simulink model "Mdl_DLR"  (R2021b)
settings: Solver=FixedStepAuto  StartTime=0.0  StopTime=10.0  FixedStep=DT_s  RelTol=1e-3
values from neighbouring files (symbols this model uses):
  BEMTPitchMax_deg = -30.0    [DD_Mdl.sldd]    (also in initRotorsimulationNREL5MW.m = -30)
  BladeLength_m = 61.5    [DD_Mdl.sldd]    (also in initRotorsimulationNREL5MW.m)
  BladeMass_kg = 17740.0    [DD_Mdl.sldd]    (also in initRotorsimulationNREL5MW.m = 17740)
  BladePitchMax_deg = 0.0    [DD_Mdl.sldd]    (also in initRotorsimulationNREL5MW.m = 0)
  BladePitchrateNorm_degpers = 3.0    [DD_Mdl.sldd]    (also in initRotorsimulationNREL5MW.m = 3)
  BladePitchrateStop_degpers = 9.0    [DD_Mdl.sldd]    (also in initRotorsimulationNREL5MW.m = 9)
  BladePitchStart_deg = -85.0    [DD_Mdl.sldd]    (also in initRotorsimulationNREL5MW.m = -85)
  BladePrecone_deg = 2.5    [DD_Mdl.sldd]    (also in initRotorsimulationNREL5MW.m)
  BladeTwist_deg = 13.308 13.308 13.308 13.308 13.308 13.308 13.308 13.308 13.308 13.308 13.308 13.308 13.181 12.848 12.192 11.561 11.072 10.792 10.232 9.672 9.11 8.534 7.932 7.321 6.711 6.122 5.546 4.971 4.401 3.834 3.332 2.89 2.503 2.116 1.73 1.342 0.954 0.76 0.574 0.404 0.319 0.253 0.216 0.178 0.14 0.101 0.062 0.023 0.0    [DD_Mdl.sldd]    (also in initRotorsimulationNREL5MW.m = [13.308 13.308 13.308 13.308 13.308 13.308 13.308 13.308 13.)
  cperR = 0.054 0.054 0.056 0.058 0.06 0.061 0.063 0.065 0.067 0.069 0.07 0.072 0.073 0.073 0.073 0.074 0.073 0.072 0.071 0.069 0.068 0.066 0.064 0.062 0.06 0.058 0.056 0.054 0.052 0.05 0.049 0.047 0.045 0.043 0.041 0.039 0.037 0.036 0.035 0.033 0.032 0.03 0.028 0.026 0.024 0.022 0.02 0.018 0.017    [DD_Mdl.sldd]    (also in initRotorsimulationNREL5MW.m = [0.054 0.054 0.056 0.058 0.060 0.061 0.063 0.065 0.067 0.069)
  Cut_OffWindSpeed_mpers = 25.0    [DD_Mdl.sldd]    (also in initRotorsimulationNREL5MW.m = 25)
  DownwashCorrection = 0.26    [DD_Mdl.sldd]    (also in initRotorsimulationNREL5MW.m)
  DownwashModelSwitch = 3.0    [DD_Mdl.sldd]    (also in initRotorsimulationNREL5MW.m = 3)
  drperR = 0.024 0.003 0.016 0.016 0.016 0.016 0.016 0.016 0.016 0.016 0.016 0.016 0.016 0.016 0.016 0.016 0.016 0.016 0.032 0.032 0.032 0.032 0.032 0.032 0.032 0.032 0.032 0.032 0.032 0.032 0.032 0.032 0.032 0.032 0.032 0.032 0.032 0.016 0.016 0.016 0.008 0.008 0.008 0.008 0.008 0.008 0.008 0.008 0.005    [DD_Mdl.sldd]    (also in initRotorsimulationNREL5MW.m = [0.024 0.003 0.016 0.016 0.016 0.016 0.016 0.016 0.016 0.016)
  DT = 0.008    [DD_LPV.sldd]    (also in DD_Mdl.sldd)
  DT_s = 0.008    [DD_Mdl.sldd]    (also in initRotorsimulationNREL5MW.m = 0.01)
  g_mpers_2 = 9.81    [DD_Mdl.sldd]    (also in initRotorsimulationNREL5MW.m)
  GeneratorEfficiency = 0.944    [DD_Mdl.sldd]    (also in initRotorsimulationNREL5MW.m)
  GeneratorOptimalModeGain_Nmper_radpers2 = 2128600    [initRotorsimulationNREL5MW.m]
  HubRadius_m = 1.5    [DD_Mdl.sldd]    (also in initRotorsimulationNREL5MW.m)
  Ki = 0.3    [initRotorsimulationNREL5MW.m]
  Kp = 0.1    [initRotorsimulationNREL5MW.m]
  mpermBl = 0.058 0.008 0.044 0.043 0.042 0.034 0.026 0.024 0.023 0.022 0.023 0.024 0.024 0.023 0.022 0.02 0.02 0.02 0.039 0.038 0.037 0.036 0.034 0.033 0.03 0.029 0.028 0.025 0.023 0.021 0.019 0.018 0.016 0.015 0.012 0.011 0.01 0.005 0.004 0.004 0.002 0.002 0.002 0.002 0.001 0.001 0.001 0.0 0.0    [DD_Mdl.sldd]    (also in initRotorsimulationNREL5MW.m = [0.058 0.008 0.044 0.043 0.042 0.034 0.026 0.024 0.023 0.022)
  nBl = 3.0    [DD_Mdl.sldd]    (also in initRotorsimulationNREL5MW.m = 3)
  nR = 49.0    [DD_Mdl.sldd]    (also in initRotorsimulationNREL5MW.m = length(drperR))
  Overhang_m = 5.0    [DD_Mdl.sldd]    (also in initRotorsimulationNREL5MW.m = 5)
  RatedOmega_RPM = 12.1    [DD_Mdl.sldd]    (also in initRotorsimulationNREL5MW.m)
  RatedWindSpeed_mpers = 11.4    [DD_Mdl.sldd]    (also in initRotorsimulationNREL5MW.m)
  rho_kgperm3 = 1.225    [DD_Mdl.sldd]    (also in initRotorsimulationNREL5MW.m)
  rperR = 0.024 0.027 0.043 0.059 0.075 0.09 0.106 0.122 0.138 0.154 0.17 0.186 0.202 0.217 0.233 0.249 0.265 0.281 0.313 0.344 0.376 0.408 0.44 0.471 0.503 0.535 0.567 0.598 0.63 0.662 0.694 0.725 0.757 0.789 0.821 0.852 0.884 0.9 0.916 0.932 0.94 0.948 0.956 0.963 0.971 0.979 0.987 0.995 1.0    [DD_Mdl.sldd]    (also in initRotorsimulationNREL5MW.m = [0.024 0.027 0.043 0.059 0.075 0.090 0.106 0.122 0.138 0.154)
  Shafttilt_deg = 5.0    [DD_Mdl.sldd]    (also in initRotorsimulationNREL5MW.m = 5)
  TipSpeedLoss = 0.0    [DD_Mdl.sldd]    (also in initRotorsimulationNREL5MW.m = 0)
  TowerDamOnperoff = 0.0    [DD_Mdl.sldd]    (also in initRotorsimulationNREL5MW.m = 0)
  TowerDragCoefficient = 0.35    [DD_Mdl.sldd]    (also in initRotorsimulationNREL5MW.m)
  TowerRadius_m = 1.935    [DD_Mdl.sldd]    (also in initRotorsimulationNREL5MW.m)
  wecs = 3.0    [DD_Mdl.sldd]    (also in DD_Mdl1.sldd = 3.0
libraries: simulink x3
(part 1 of 2)
settings Model: DataDictionary=DD_Mdl.sldd  Creator=ditt_aj  LastModifiedBy=ditt_aj
settings SolverCC: AlgebraicLoopSolver=TrustRegion
settings DebuggingCC: SFMachineParentedDataDiag=warning

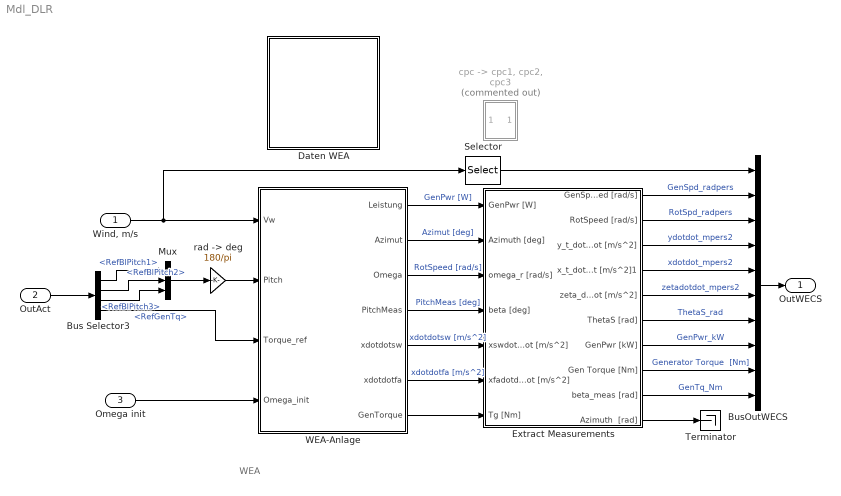
== system Mdl_DLR ==
  note: WEA
  "Wind, m/s" : Inport
  OutAct : Inport  Port=2  OutDataTypeStr=Bus: slBus2
  Omega init : Inport  Port=3
  Bus Selector3 : BusSelector  OutputSignals=RefBlPitch1,RefBlPitch2,RefBlPitch3,RefGenTq
  BusOutWECS : BusCreator  Inputs=10  OutDataTypeStr=Bus: slBus1
  Daten WEA : Subsystem
  Extract Measurements : Subsystem
  Mux : Mux  Inputs=3
  Selector : Selector  InputPortWidth=3  IndexOptions=Index vector (dialog)  Indices=1  OutputSizes=1
  Terminator : Terminator
  WEA-Anlage : Subsystem
  "cpc -> cpc1, cpc2, cpc3" : Subsystem  Commented=on
  "rad -> deg" : Gain  Gain=180/pi
  OutWECS : Outport  OutDataTypeStr=Bus: slBus1
  wires:
  WEA-Anlage/3(Omega) -> Extract Measurements/3("omega_r [rad/s] ")  "RotSpeed [rad/s]"
  WEA-Anlage/2(Azimut) -> Extract Measurements/2(Azimuth [deg])  "Azimut [deg]"
  WEA-Anlage/1(Leistung) -> Extract Measurements/1("GenPwr [W] ")  "GenPwr [W]"
  Omega init/1 -> WEA-Anlage/4(Omega_init)
  WEA-Anlage/4(PitchMeas) -> Extract Measurements/4(beta [deg])  "PitchMeas [deg]"
  WEA-Anlage/5("xdotdotsw ") -> Extract Measurements/5(xswdotdot [m/s^2])  "xdotdotsw [m/s^2]"
  WEA-Anlage/6("xdotdotfa ") -> Extract Measurements/6(xfadotdot [m/s^2])  "xdotdotfa [m/s^2]"
  WEA-Anlage/7(GenTorque) -> Extract Measurements/7(Tg [Nm])
  OutAct/1 -> Bus Selector3/1
  Bus Selector3/4 -> WEA-Anlage/3(Torque_ref)  "<RefGenTq>"
  BusOutWECS/1 -> OutWECS/1
  Extract Measurements/1("GenSpeed [rad/s] ") -> BusOutWECS/2  "GenSpd_radpers"
  Extract Measurements/2(" RotSpeed [rad/s]") -> BusOutWECS/3  "RotSpd_radpers"
  Extract Measurements/3(y_t_dotdot [m/s^2]) -> BusOutWECS/4  "ydotdot_mpers2"
  Extract Measurements/4(x_t_dotdot [m/s^2]1) -> BusOutWECS/5  "xdotdot_mpers2"
  Extract Measurements/5(zeta_dotdot [m/s^2]) -> BusOutWECS/6  "zetadotdot_mpers2"
  Extract Measurements/6(ThetaS [rad]) -> BusOutWECS/7  "ThetaS_rad"
  Extract Measurements/7(GenPwr [kW]) -> BusOutWECS/8  "GenPwr_kW"
  Extract Measurements/8("Gen Torque [Nm]  ") -> BusOutWECS/9  "Generator Torque  [Nm]"
  Extract Measurements/9(beta_meas [rad]) -> BusOutWECS/10  "GenTq_Nm"
  Extract Measurements/10(Azimuth  [rad]) -> Terminator/1
  Mux/1 -> "rad -> deg"/1
  Bus Selector3/1 -> Mux/1  "<RefBlPitch1>"
  Bus Selector3/2 -> Mux/2  "<RefBlPitch2>"
  Bus Selector3/3 -> Mux/3  "<RefBlPitch3>"
  "Wind, m/s"/1 -> WEA-Anlage/1(Vw), Selector/1
  "rad -> deg"/1 -> WEA-Anlage/2(Pitch)
  Selector/1 -> BusOutWECS/1

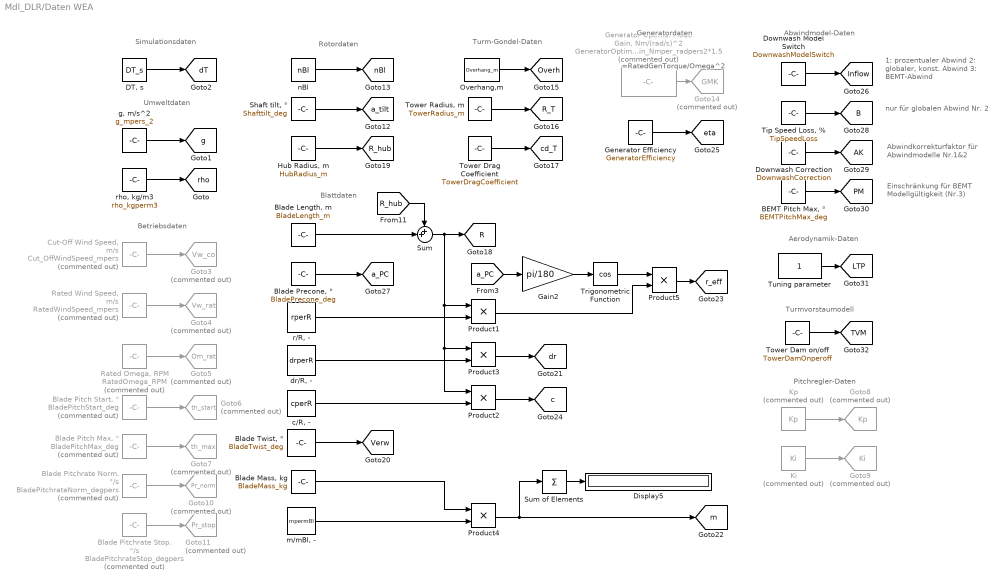
== system Mdl_DLR/Daten WEA ==
  note: Aerodynamik-Daten
  note: Simulationsdaten
  note: Abwindkorrekturfaktor für
      | Abwindmodelle Nr.1&2
  note: Umweltdaten
  note: =RatedGenTorque/Omega^2
  note: Generatordaten
  note: Pitchregler-Daten
  note: Rotordaten
  note: Einschränkung für BEMT
      | Modellgültigkeit (Nr.3)
  note: Betriebsdaten
  note: Abwindmodel-Daten
  note: Turm-Gondel-Daten
  note: nur für globalen Abwind Nr. 2
  note: 1: prozentualer Abwind
      | 2: globaler, konst. Abwind
      | 3: BEMT-Abwind
  note: Turmvorstaumodell
  note: Blattdaten
  "BEMT Pitch Max, °" : Constant  Value=BEMTPitchMax_deg
  "Blade Length, m" : Constant  Value=BladeLength_m
  "Blade Mass, kg" : Constant  Value=BladeMass_kg
  "Blade Pitch Max, °" : Constant  Commented=on  Value=BladePitchMax_deg
  "Blade Pitch Start, °" : Constant  Commented=on  Value=BladePitchStart_deg
  Blade Pitchrate Norm. °/s : Constant  Commented=on  Value=BladePitchrateNorm_degpers
  Blade Pitchrate Stop. °/s : Constant  Commented=on  Value=BladePitchrateStop_degpers
  "Blade Precone, °" : Constant  Value=BladePrecone_deg
  "Blade Twist, °" : Constant  Value=BladeTwist_deg
  "Cut-Off Wind Speed, m/s" : Constant  Commented=on  Value=Cut_OffWindSpeed_mpers
  "DT, s" : Constant  Value=DT_s
  Display5 : Display
  Downwash Correction : Constant  Value=DownwashCorrection
  Downwash Model Switch : Constant  Value=DownwashModelSwitch
  Gain2 : Gain  Gain=pi/180
  Generator Efficiency : Constant  Value=GeneratorEfficiency
  "Generator Optimal Mode Gain, Nm/(rad/s)^2" : Constant  Commented=on  Value=GeneratorOptimalModeGain_Nmper_radpers2*1.5
  Goto10 : Goto  Commented=on  GotoTag=Pr_norm  TagVisibility=global
  Goto11 : Goto  Commented=on  GotoTag=Pr_stop  TagVisibility=global
  Goto14 : Goto  Commented=on  GotoTag=GMK  TagVisibility=global
  Goto3 : Goto  Commented=on  GotoTag=Vw_co  TagVisibility=global
  Goto4 : Goto  Commented=on  GotoTag=Vw_rat  TagVisibility=global
  Goto5 : Goto  Commented=on  GotoTag=Om_rat  TagVisibility=global
  Goto6 : Goto  Commented=on  GotoTag=th_start  TagVisibility=global
  Goto7 : Goto  Commented=on  GotoTag=th_max  TagVisibility=global
  Goto8 : Goto  Commented=on  GotoTag=Kp  TagVisibility=global
  Goto9 : Goto  Commented=on  GotoTag=Ki  TagVisibility=global
  "Hub Radius, m" : Constant  Value=HubRadius_m
  Ki : Constant  Commented=on  Value=Ki
  Kp : Constant  Commented=on  Value=Kp
  Overhang,m : Constant  Value=Overhang_m
  Product{1..5} (5 alike) : Product  RndMeth=Zero
  "Rated Omega, RPM" : Constant  Commented=on  Value=RatedOmega_RPM
  "Rated Wind Speed, m/s" : Constant  Commented=on  Value=RatedWindSpeed_mpers
  "Shaft tilt, °" : Constant  Value=Shafttilt_deg
  Sum : Sum  Inputs=++|
  Sum of Elements : Sum  Inputs=+
  "Tip Speed Loss, %" : Constant  Value=TipSpeedLoss
  Tower Dam on/off : Constant  Value=TowerDamOnperoff
  Tower Drag Coefficient : Constant  Value=TowerDragCoefficient
  "Tower Radius, m" : Constant  Value=TowerRadius_m
  Trigonometric Function : Trigonometry  Operator=cos
  Tuning parameter : Constant
  "c/R, -" : Constant  Value=cperR
  "dr/R, -" : Constant  Value=drperR
  "g, m/s^2" : Constant  Value=g_mpers_2
  "m/mBl, - " : Constant  Value=mpermBl
  nBl : Constant  Value=nBl
  "r/R, -" : Constant  Value=rperR
  "rho, kg/m3" : Constant  Value=rho_kgperm3
  tag scope: AK=global, B=global, Inflow=global, LTP=global, Overh=global, PM=global, R=global, R_T=global, R_hub=global, TVM=global, Verw=global, a_PC=global, a_tilt=global, c=global, cd_T=global, dT=global, dr=global, eta=global, g=global, m=global, nBl=global, r_eff=global, rho=global
  wires:
  Tower Dam on/off/1 -> [TVM]
  Generator Efficiency/1 -> [eta]
  "Blade Precone, °"/1 -> [a_PC]
  "Tower Radius, m"/1 -> [R_T]
  "r/R, -"/1 -> Product1/2
  Downwash Correction/1 -> [AK]
  "DT, s"/1 -> [dT]
  "Blade Pitch Max, °"/1 -> Goto7/1
  [R_hub] -> Sum/1
  "BEMT Pitch Max, °"/1 -> [PM]
  [a_PC] -> Gain2/1
  "Tip Speed Loss, %"/1 -> [B]
  Tuning parameter/1 -> [LTP]
  "g, m/s^2"/1 -> [g]
  "Blade Mass, kg"/1 -> Product4/1
  "Rated Wind Speed, m/s"/1 -> Goto4/1
  Blade Pitchrate Stop. °/s/1 -> Goto11/1
  Sum/1 -> [R], Product1/1, Product3/1, Product2/1
  Downwash Model Switch/1 -> [Inflow]
  Product1/1 -> Product5/2
  Sum of Elements/1 -> Display5/1
  "c/R, -"/1 -> Product2/2
  "Blade Length, m"/1 -> Sum/2
  "Hub Radius, m"/1 -> [R_hub]
  "m/mBl, - "/1 -> Product4/2
  "Shaft tilt, °"/1 -> [a_tilt]
  Product4/1 -> [m], Sum of Elements/1
  Product2/1 -> [c]
  "Blade Twist, °"/1 -> [Verw]
  Tower Drag Coefficient/1 -> [cd_T]
  "dr/R, -"/1 -> Product3/2
  Product3/1 -> [dr]
  Product5/1 -> [r_eff]
  "Blade Pitch Start, °"/1 -> Goto6/1
  Gain2/1 -> Trigonometric Function/1
  "Rated Omega, RPM"/1 -> Goto5/1
  Kp/1 -> Goto8/1
  nBl/1 -> [nBl]
  "Cut-Off Wind Speed, m/s"/1 -> Goto3/1
  Ki/1 -> Goto9/1
  Blade Pitchrate Norm. °/s/1 -> Goto10/1
  "Generator Optimal Mode Gain, Nm/(rad/s)^2"/1 -> Goto14/1
  Trigonometric Function/1 -> Product5/1
  Overhang,m/1 -> [Overh]
  "rho, kg/m3"/1 -> [rho]

== system Mdl_DLR/Extract Measurements ==
  "GenPwr [W] " : Inport
  Azimuth [deg] : Inport  Port=2
  "omega_r [rad/s] " : Inport  Port=3
  beta [deg] : Inport  Port=4
  xswdotdot [m/s^2] : Inport  Port=5
  xfadotdot [m/s^2] : Inport  Port=6
  Tg [Nm] : Inport  Port=7
  "Azimuth: deg -> rad" : Gain  Gain=pi/180
  Demux : Demux  Outputs=3
  Gain6 : Gain  Gain=wecs.Ng
  "GenPwr: W -> kW1" : Gain  Gain=1/1000
  Ground1 : Ground
  "Pitch: deg -> rad" : Gain  Gain=pi/180
  Sum : Sum  Inputs=+-
  Terminator : Terminator
  Terminator1 : Terminator
  "GenSpeed [rad/s] " : Outport  VectorParamsAs1DForOutWhenUnconnected=off
  " RotSpeed [rad/s]" : Outport  Port=2  VectorParamsAs1DForOutWhenUnconnected=off
  y_t_dotdot [m/s^2] : Outport  Port=3  VectorParamsAs1DForOutWhenUnconnected=off
  x_t_dotdot [m/s^2]1 : Outport  Port=4  VectorParamsAs1DForOutWhenUnconnected=off
  zeta_dotdot [m/s^2] : Outport  Port=5  VectorParamsAs1DForOutWhenUnconnected=off
  ThetaS [rad] : Outport  Port=6  VectorParamsAs1DForOutWhenUnconnected=off
  GenPwr [kW] : Outport  Port=7  VectorParamsAs1DForOutWhenUnconnected=off
  "Gen Torque [Nm]  " : Outport  Port=8  VectorParamsAs1DForOutWhenUnconnected=off
  beta_meas [rad] : Outport  Port=9  VectorParamsAs1DForOutWhenUnconnected=off
  Azimuth  [rad] : Outport  Port=10  VectorParamsAs1DForOutWhenUnconnected=off
  wires:
  xfadotdot [m/s^2]/1 -> y_t_dotdot [m/s^2]/1  "y_t_dotdot"
  Gain6/1 -> "GenSpeed [rad/s] "/1  "omega_g [rad/s]"
  Tg [Nm]/1 -> "Gen Torque [Nm]  "/1
  Sum/1 -> ThetaS [rad]/1  "rad"
  "omega_r [rad/s] "/1 -> " RotSpeed [rad/s]"/1, Sum/2, Sum/1, Gain6/1  "GenSpeed [rad/s] LSS"
  Ground1/1 -> zeta_dotdot [m/s^2]/1  "zeta_dotdot"
  xswdotdot [m/s^2]/1 -> x_t_dotdot [m/s^2]1/1  "y_t_dotdot"
  beta [deg]/1 -> "Pitch: deg -> rad"/1  "Pitch [deg]"
  "GenPwr [W] "/1 -> "GenPwr: W -> kW1"/1  "Gen Pwr [W]"
  "GenPwr: W -> kW1"/1 -> GenPwr [kW]/1  "Generator Power [kW]"
  "Azimuth: deg -> rad"/1 -> Azimuth  [rad]/1  "Azimuth [rad]"
  Azimuth [deg]/1 -> "Azimuth: deg -> rad"/1  "Azimuth [deg]"
  "Pitch: deg -> rad"/1 -> Demux/1  "Pitch [rad]"
  Demux/3 -> Terminator/1
  Demux/2 -> Terminator1/1
  Demux/1 -> beta_meas [rad]/1

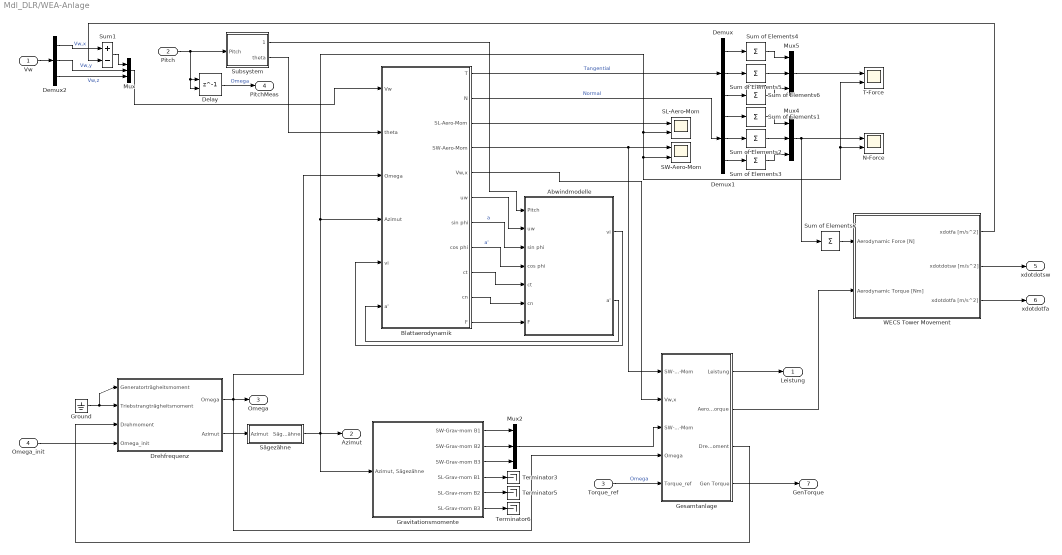
== system Mdl_DLR/WEA-Anlage ==
  Vw : Inport
  Pitch : Inport  Port=2
  Torque_ref : Inport  Port=3
  Omega_init : Inport  Port=4
  Abwindmodelle : Subsystem
  Blattaerodynamik : Subsystem
  Delay : Delay  DelayLength=1  InitialConditionSource=Input port
      settings: InputPortMap=u0,p4
  Demux : Demux  Outputs=3
  Demux1 : Demux  Outputs=3
  Demux2 : Demux  Outputs=3
  Drehfrequenz : Subsystem
  Gesamtanlage : Subsystem
  Gravitationsmomente : Subsystem
  Ground : Ground
  Mux{,2,4..5} (4 alike) : Mux  Inputs=3
  N-Force : Scope  NumInputPorts=2
  SL-Aero-Mom : Scope  NumInputPorts=2
  SW-Aero-Mom : Scope  NumInputPorts=2
  Subsystem : Subsystem
  Sum of Elements{1..7} (7 alike) : Sum  Inputs=+
  Sum1 : Sum  Inputs=+-
  Sägezähne : Subsystem
  T-Force : Scope  NumInputPorts=2
  Terminator3 : Terminator
  Terminator5 : Terminator
  Terminator6 : Terminator
  WECS Tower Movement : Subsystem
  Leistung : Outport  VectorParamsAs1DForOutWhenUnconnected=off
  Azimut : Outport  Port=2  VectorParamsAs1DForOutWhenUnconnected=off
  Omega : Outport  Port=3  VectorParamsAs1DForOutWhenUnconnected=off
  PitchMeas : Outport  Port=4  VectorParamsAs1DForOutWhenUnconnected=off
  "xdotdotsw " : Outport  Port=5  VectorParamsAs1DForOutWhenUnconnected=off
  "xdotdotfa " : Outport  Port=6  VectorParamsAs1DForOutWhenUnconnected=off
  GenTorque : Outport  Port=7  VectorParamsAs1DForOutWhenUnconnected=off
  wires:
  Blattaerodynamik/1(T) -> Demux/1  "Tangential"
  Blattaerodynamik/2(N) -> Demux1/1  "Normal"
  Sägezähne/1(Sägezähne) -> Gravitationsmomente/1("Azimut, Sägezähne"), Blattaerodynamik/4(Azimut), SL-Aero-Mom/2, SW-Aero-Mom/2, N-Force/2, T-Force/2, Azimut/1
  Drehfrequenz/2(Azimut) -> Sägezähne/1(Azimut)
  Blattaerodynamik/4(SW-Aero-Mom) -> Gesamtanlage/1(SW-Aero-Mom), SW-Aero-Mom/1
  Blattaerodynamik/3(SL-Aero-Mom) -> SL-Aero-Mom/1
  Gravitationsmomente/1(SW-Grav-mom B1) -> Mux2/1
  Gravitationsmomente/2(SW-Grav-mom B2) -> Mux2/2
  Gravitationsmomente/3(SW-Grav-mom B3) -> Mux2/3
  Abwindmodelle/1(vi) -> Blattaerodynamik/5(vi)
  Blattaerodynamik/8(cos phi) -> Abwindmodelle/4(cos phi)  "a'"
  Blattaerodynamik/7(sin phi) -> Abwindmodelle/3(sin phi)  "a"
  Blattaerodynamik/10(cn) -> Abwindmodelle/6(cn)
  Blattaerodynamik/9(ct) -> Abwindmodelle/5(ct)
  Abwindmodelle/2(a') -> Blattaerodynamik/6(a')
  Subsystem/2(theta) -> Blattaerodynamik/2(theta)
  Blattaerodynamik/11(F) -> Abwindmodelle/7(F)
  Gravitationsmomente/4(SL-Grav-mom B1) -> Terminator3/1
  Gravitationsmomente/6(SL-Grav-mom B3) -> Terminator6/1
  Gravitationsmomente/5(SL-Grav-mom B2) -> Terminator5/1
  Drehfrequenz/1(Omega) -> Gesamtanlage/4(Omega), Omega/1, Blattaerodynamik/3(Omega)
  Mux2/1 -> Gesamtanlage/3(SW-Grav-Mom)
  Gesamtanlage/1(Leistung) -> Leistung/1
  Gesamtanlage/3(Drehmoment) -> Drehfrequenz/3(Drehmoment)
  Demux1/1 -> Sum of Elements1/1
  Demux1/2 -> Sum of Elements2/1
  Demux1/3 -> Sum of Elements3/1
  Sum of Elements1/1 -> Mux4/1
  Sum of Elements2/1 -> Mux4/2
  Demux/1 -> Sum of Elements4/1
  Demux/2 -> Sum of Elements5/1
  Demux/3 -> Sum of Elements6/1
  Sum of Elements4/1 -> Mux5/1
  Sum of Elements6/1 -> Mux5/3
  Sum of Elements5/1 -> Mux5/2
  Mux5/1 -> T-Force/1
  Blattaerodynamik/5(Vw,x) -> Gesamtanlage/2(Vw,x)
  Blattaerodynamik/6(" uw") -> Abwindmodelle/2(uw)
  Subsystem/1(CPC +IPC) -> Abwindmodelle/1(Pitch)
  Ground/1 -> Drehfrequenz/1(Generatorträgheitsmoment), Drehfrequenz/2(Triebstrangträgheitsmoment)
  Sum of Elements3/1 -> Mux4/3
  Pitch/1 -> Delay/2, Delay/1, Subsystem/1(Pitch)
  Omega_init/1 -> Drehfrequenz/4(Omega_init)
  Delay/1 -> PitchMeas/1  "Omega"
  Mux4/1 -> N-Force/1, Sum of Elements7/1
  Sum of Elements7/1 -> WECS Tower Movement/1(Aerodynamic Force [N])
  Torque_ref/1 -> Gesamtanlage/5(Torque_ref)  "Omega"
  WECS Tower Movement/3(xdotdotfa [m/s^2]) -> "xdotdotfa "/1
  WECS Tower Movement/2(xdotdotsw [m/s^2]) -> "xdotdotsw "/1
  WECS Tower Movement/1(xdotfa [m/s^2]) -> Sum1/2
  Vw/1 -> Demux2/1
  Demux2/1 -> Sum1/1  "Vw,x"
  Sum1/1 -> Mux/1
  Demux2/2 -> Mux/2  "Vw,y"
  Demux2/3 -> Mux/3  "Vw,z"
  Mux/1 -> Blattaerodynamik/1(Vw)
  Gesamtanlage/2(Aero Torque) -> WECS Tower Movement/2(Aerodynamic Torque [Nm])
  Gesamtanlage/4(Gen Torque) -> GenTorque/1

== system Mdl_DLR/cpc -> cpc1, cpc2, cpc3 ==
  beta_ref [rad] : Inport
  Mux : Mux  Inputs=3
  "rad -> deg" : Gain  Gain=180/pi
  "Pitch_ref123 [deg] " : Outport  VectorParamsAs1DForOutWhenUnconnected=off
  wires:
  beta_ref [rad]/1 -> "rad -> deg"/1
  Mux/1 -> "Pitch_ref123 [deg] "/1
  "rad -> deg"/1 -> ?

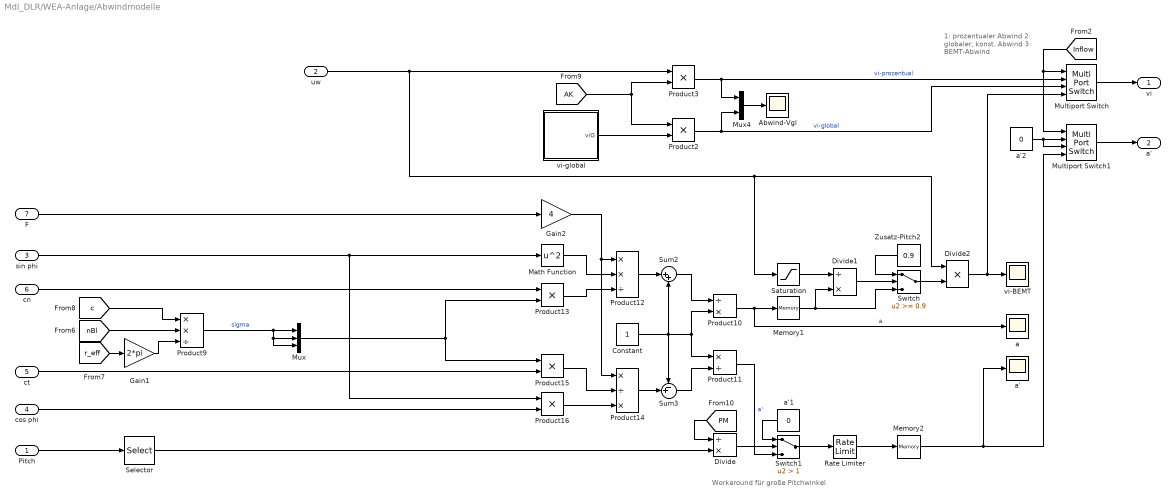
== system Mdl_DLR/WEA-Anlage/Abwindmodelle ==
  note: Workaround für große Pitchwinkel
  note: 1: prozentualer Abwind
      | 2: globaler, konst. Abwind
      | 3: BEMT-Abwind
  Pitch : Inport
  uw : Inport  Port=2
  sin phi : Inport  Port=3
  cos phi : Inport  Port=4
  ct : Inport  Port=5
  cn : Inport  Port=6
  F : Inport  Port=7
  " a " : Scope
  " a' " : Scope
  Abwind-Vgl : Scope
  Constant : Constant
  Divide : Product  Inputs=/*
  Divide1 : Product  Inputs=/*
  Divide2 : Product
  Gain1 : Gain  Gain=2*pi
  Gain2 : Gain  Gain=4
  Math Function : Math  Operator=square  SignedPower=on  SaturateOnIntegerOverflow=on
  Memory1 : Memory
  Memory2 : Memory
  Multiport Switch : MultiPortSwitch  RndMeth=Nearest
  Multiport Switch1 : MultiPortSwitch  RndMeth=Nearest
  Mux : Mux  Inputs=3
  Mux4 : Mux  Inputs=2
  Product10 : Product  Inputs=/*  RndMeth=Zero
  Product11 : Product  Inputs=*/  RndMeth=Zero
  Product12 : Product  Inputs=**/  RndMeth=Zero
  Product{2..3,13,15..16} (5 alike) : Product  RndMeth=Zero
  Product14 : Product  Inputs=*/*  RndMeth=Zero
  Product9 : Product  Inputs=**/  RndMeth=Zero
  Rate Limiter : RateLimiter  SampleTimeMode=inherited
  Saturation : Saturate  UpperLimit=inf  LowerLimit=0.01
  Selector : Selector  InputPortWidth=3  IndexOptions=Index vector (dialog)  Indices=1  OutputSizes=1
  Sum2 : Sum  Inputs=|++
  Sum3 : Sum  Inputs=-+|
  Switch : Switch  Threshold=0.9
  Switch1 : Switch  Criteria=u2 > Threshold  Threshold=1
  Zusatz-Pitch2 : Constant  Value=0.9
  a'1 : Constant  Value=0
  a'2 : Constant  Value=0
  vi-BEMT : Scope
  vi-global : Subsystem
  vi : Outport  VectorParamsAs1DForOutWhenUnconnected=off
  a' : Outport  Port=2  VectorParamsAs1DForOutWhenUnconnected=off
  wires:
  vi-global/1(viG) -> Product2/2
  Product2/1 -> Mux4/2, Multiport Switch/3  "vi-global"
  Saturation/1 -> Divide1/1
  Zusatz-Pitch2/1 -> Switch/1
  Memory1/1 -> Divide1/2, Switch/3
  Switch/1 -> Divide2/2
  Divide1/1 -> Switch/2
  Divide2/1 -> vi-BEMT/1, Multiport Switch/4
  [Inflow] -> Multiport Switch/1, Multiport Switch1/1
  Mux4/1 -> Abwind-Vgl/1
  Product3/1 -> Mux4/1, Multiport Switch/2  "vi-prozentual"
  uw/1 -> Saturation/1, Divide2/1, Product3/1
  Multiport Switch/1 -> vi/1
  cos phi/1 -> Product16/2
  sin phi/1 -> Math Function/1, Product16/1
  Constant/1 -> Sum3/1, Sum2/2, Product11/1, Product10/2
  Math Function/1 -> Product12/2
  Product13/1 -> Product12/3
  cn/1 -> Product13/1
  Product16/1 -> Product14/3
  ct/1 -> Product15/2
  Product12/1 -> Sum2/1
  Product14/1 -> Sum3/2
  Sum2/1 -> Product10/1
  Sum3/1 -> Product11/2
  Product10/1 -> Memory1/1, " a "/1  "a"
  Product11/1 -> Switch1/3  "a'"
  [c] -> Product9/1
  [nBl] -> Product9/2
  [r_eff] -> Gain1/1
  Gain1/1 -> Product9/3
  a'2/1 -> Multiport Switch1/2, Multiport Switch1/3
  Multiport Switch1/1 -> a'/1
  F/1 -> Gain2/1
  Gain2/1 -> Product12/1, Product14/1
  Product15/1 -> Product14/2
  Pitch/1 -> Selector/1
  Divide/1 -> Switch1/2
  a'1/1 -> Switch1/1
  [PM] -> Divide/1
  Switch1/1 -> Rate Limiter/1
  Rate Limiter/1 -> Memory2/1
  Memory2/1 -> " a' "/1, Multiport Switch1/4
  [AK] -> Product3/2, Product2/1
  Selector/1 -> Divide/2
  Product9/1 -> Mux/3, Mux/2, Mux/1  "sigma"
  Mux/1 -> Product15/1, Product13/2

== system Mdl_DLR/WEA-Anlage/Blattaerodynamik ==
  Vw : Inport
  theta : Inport  Port=2
  Omega : Inport  Port=3
  Azimut : Inport  Port=4
  vi : Inport  Port=5
  a' : Inport  Port=6
  Anströmung : Subsystem
  Beiwerte1 : Subsystem
  Beiwerte2 : Subsystem
  Blattbiegemomente : Subsystem
  Gain5 : Gain  Gain=pi/180
  Komponenten für BEMT : Subsystem
  Normal-/Tangentialkraft : Subsystem
  Tip&Hub-Loss-Faktor : Subsystem
  T : Outport  VectorParamsAs1DForOutWhenUnconnected=off
  N : Outport  Port=2  VectorParamsAs1DForOutWhenUnconnected=off
  SL-Aero-Mom : Outport  Port=3  VectorParamsAs1DForOutWhenUnconnected=off
  SW-Aero-Mom : Outport  Port=4  VectorParamsAs1DForOutWhenUnconnected=off
  Vw,x : Outport  Port=5  VectorParamsAs1DForOutWhenUnconnected=off
  " uw" : Outport  Port=6  VectorParamsAs1DForOutWhenUnconnected=off
  sin phi : Outport  Port=7  VectorParamsAs1DForOutWhenUnconnected=off
  cos phi : Outport  Port=8  VectorParamsAs1DForOutWhenUnconnected=off
  ct : Outport  Port=9  VectorParamsAs1DForOutWhenUnconnected=off
  cn : Outport  Port=10  VectorParamsAs1DForOutWhenUnconnected=off
  F : Outport  Port=11  VectorParamsAs1DForOutWhenUnconnected=off
  wires:
  Beiwerte2/1(cl) -> Normal-/Tangentialkraft/1(cl)
  Beiwerte2/2(cd) -> Normal-/Tangentialkraft/2(cd)
  Anströmung/2(phi) -> Normal-/Tangentialkraft/3("phi, rad")
  Anströmung/3(V^2) -> Normal-/Tangentialkraft/4(V^2)
  Vw/1 -> Anströmung/2(Vw)
  Omega/1 -> Anströmung/4(Omega)
  Normal-/Tangentialkraft/1(T) -> T/1, Blattbiegemomente/1(T)
  Normal-/Tangentialkraft/2(N) -> N/1, Blattbiegemomente/2(N)
  Komponenten für BEMT/1(sin phi) -> sin phi/1, Tip&Hub-Loss-Faktor/1(sin phi)
  theta/1 -> Anströmung/1(theta)
  vi/1 -> Anströmung/3(vi)
  Komponenten für BEMT/3(ct) -> ct/1
  Komponenten für BEMT/4(cn) -> cn/1
  a'/1 -> Anströmung/5(a')
  Anströmung/1(alf_eff) -> Beiwerte2/1("alf_eff, rad")
  Tip&Hub-Loss-Faktor/1(F) -> F/1
  Azimut/1 -> Gain5/1
  Gain5/1 -> Anströmung/6(Azimut)
  Anströmung/5(uw) -> " uw"/1
  Anströmung/4(Vw,x) -> Vw,x/1
  Anströmung/6(phi BEMT) -> Komponenten für BEMT/1("phi, BEMT")
  Komponenten für BEMT/2(cos phi) -> cos phi/1
  Anströmung/7(alf_eff_BEMT) -> Beiwerte1/1("alf_eff, rad")
  Beiwerte1/1(cl) -> Komponenten für BEMT/2(cl)
  Beiwerte1/2(cd) -> Komponenten für BEMT/3(cd)
  Blattbiegemomente/1(SW-Aero-Mom) -> SW-Aero-Mom/1
  Blattbiegemomente/2(SL-Aero-Mom) -> SL-Aero-Mom/1

== system Mdl_DLR/WEA-Anlage/Drehfrequenz ==
  note: Omega = Omega0 + dOm/dt*t
  note: Psi = Psi0 + Omega0*t + 1/2*dOm/dt*t^2
  note: Rotorträgheits-
      | moment
  Generatorträgheitsmoment : Inport
  Triebstrangträgheitsmoment : Inport  Port=2
  Drehmoment : Inport  Port=3
  Omega_init : Inport  Port=4
  Azimut1 : Scope
  Delay : Delay  DelayLength=1  InitialConditionSource=Input port
      settings: InputPortMap=u0,p4
  Delay1 : Delay  DelayLength=1  InitialConditionSource=Input port
      settings: InputPortMap=u0,p4
  Divide : Product  Inputs=*/
  Gain : Gain  Gain=1/2
  Gain4 : Gain  Gain=180/pi
  Math Function : Math  Operator=square  SignedPower=on  SaturateOnIntegerOverflow=on
  Math Function5 : Math  Operator=square  SignedPower=on  SaturateOnIntegerOverflow=on
  Memory2 : Memory
  Omega1 : Scope
  Product1 : Product  RndMeth=Zero
  Product2 : Product  RndMeth=Zero
  Product3 : Product  RndMeth=Zero
  Product4 : Product  Inputs=3  RndMeth=Zero
  Sum of Elements : Sum  Inputs=+
  Sum1 : Sum  Inputs=+++
  Sum2 : Sum  Inputs=++|
  Sum6 : Sum  Inputs=++|
  Sum7 : Sum  Inputs=+|+
  Trägheitsmoment : Display
      settings: Decimation=100
  Omega : Outport  VectorParamsAs1DForOutWhenUnconnected=off
  Azimut : Outport  Port=2  VectorParamsAs1DForOutWhenUnconnected=off
  wires:
  Drehmoment/1 -> Divide/1
  [dT] -> Product2/2, Product1/2, Math Function/1
  Divide/1 -> Gain/1, Product2/1  "dOm/dt"
  Sum2/1 -> Delay1/1, Delay/1, Product1/1  "Omega"
  Delay1/1 -> Sum2/1
  Product2/1 -> Sum2/2
  Sum6/1 -> Memory2/1, Azimut/1, Gain4/1  "Azimut"
  Memory2/1 -> Sum6/1
  Gain/1 -> Product3/2
  Math Function/1 -> Product3/1
  Product1/1 -> Sum7/1
  Product3/1 -> Sum7/2
  Sum7/1 -> Sum6/2
  Delay/1 -> Omega/1, Omega1/1  "Omega"
  [m] -> Product4/3
  Math Function5/1 -> Product4/2
  Product4/1 -> Sum of Elements/1
  [nBl] -> Product4/1
  [r_eff] -> Math Function5/1
  Sum of Elements/1 -> Sum1/2
  Generatorträgheitsmoment/1 -> Sum1/1
  Triebstrangträgheitsmoment/1 -> Sum1/3
  Sum1/1 -> Trägheitsmoment/1, Divide/2
  Gain4/1 -> Azimut1/1  "Azimut"
  Omega_init/1 -> Delay1/2, Delay/2

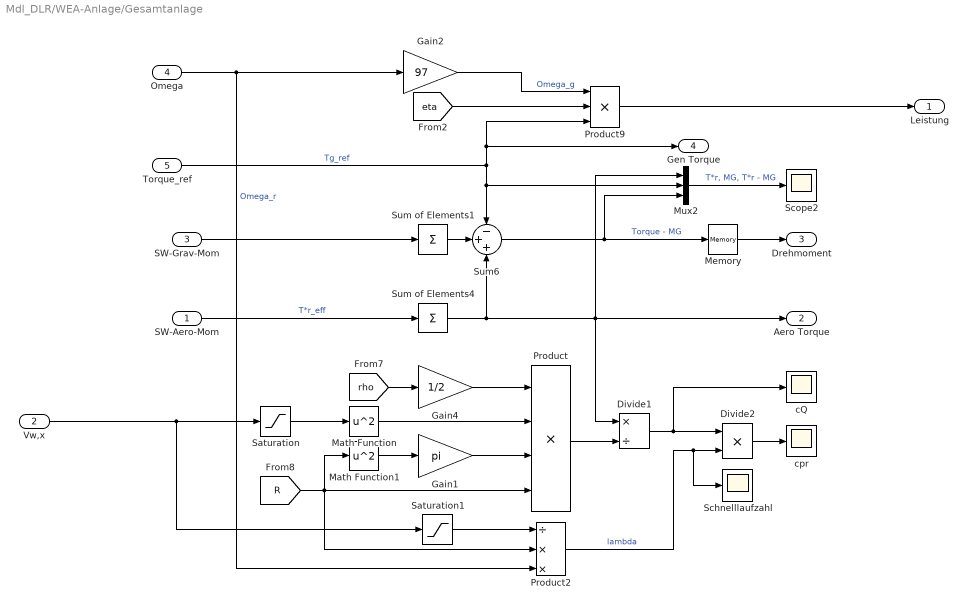
== system Mdl_DLR/WEA-Anlage/Gesamtanlage ==
  SW-Aero-Mom : Inport
  Vw,x : Inport  Port=2
  SW-Grav-Mom : Inport  Port=3
  Omega : Inport  Port=4
  Torque_ref : Inport  Port=5
  Divide1 : Product  Inputs=*/
  Divide2 : Product
  Gain1 : Gain  Gain=pi
  Gain2 : Gain  Gain=97
  Gain4 : Gain  Gain=1/2
  Math Function : Math  Operator=square  SignedPower=on  SaturateOnIntegerOverflow=on
  Math Function1 : Math  Operator=square  SignedPower=on  SaturateOnIntegerOverflow=on
  Memory : Memory
  Mux2 : Mux  Inputs=3
  Product : Product  Inputs=4  RndMeth=Zero
  Product2 : Product  Inputs=/**  RndMeth=Zero
  Product9 : Product  Inputs=3  RndMeth=Zero
  Saturation : Saturate  UpperLimit=inf  LowerLimit=0.1
  Saturation1 : Saturate  UpperLimit=inf  LowerLimit=0.1
  Schnelllaufzahl : Scope
  Scope2 : Scope
  Sum of Elements1 : Sum  Inputs=+
  Sum of Elements4 : Sum  Inputs=+
  Sum6 : Sum  Inputs=-++
  cQ : Scope
  cpr : Scope
  Leistung : Outport  VectorParamsAs1DForOutWhenUnconnected=off
  Aero Torque : Outport  Port=2  VectorParamsAs1DForOutWhenUnconnected=off
  Drehmoment : Outport  Port=3  VectorParamsAs1DForOutWhenUnconnected=off
  Gen Torque : Outport  Port=4  VectorParamsAs1DForOutWhenUnconnected=off
  wires:
  Product2/1 -> Divide2/2, Schnelllaufzahl/1  "lambda"
  Divide2/1 -> cpr/1
  Math Function/1 -> Product/2
  [R] -> Math Function1/1, Product/4, Product2/2
  Math Function1/1 -> Gain1/1
  Gain4/1 -> Product/1
  Gain1/1 -> Product/3
  Product/1 -> Divide1/2
  Divide1/1 -> Divide2/1, cQ/1
  Sum of Elements4/1 -> Sum6/3, Divide1/1, Mux2/1, Aero Torque/1
  [rho] -> Gain4/1
  Saturation/1 -> Math Function/1
  Mux2/1 -> Scope2/1  "T*r, MG, T*r - MG"
  Sum6/1 -> Mux2/3, Memory/1  "Torque - MG"
  SW-Grav-Mom/1 -> Sum of Elements1/1
  [eta] -> Product9/2
  Omega/1 -> Gain2/1, Product2/3  "Omega_r"
  SW-Aero-Mom/1 -> Sum of Elements4/1  "T*r_eff"
  Vw,x/1 -> Saturation1/1, Saturation/1
  Saturation1/1 -> Product2/1
  Sum of Elements1/1 -> Sum6/2
  Memory/1 -> Drehmoment/1
  Torque_ref/1 -> Mux2/2, Sum6/1, Gen Torque/1, Product9/3  "Tg_ref"
  Product9/1 -> Leistung/1
  Gain2/1 -> Product9/1  "Omega_g"

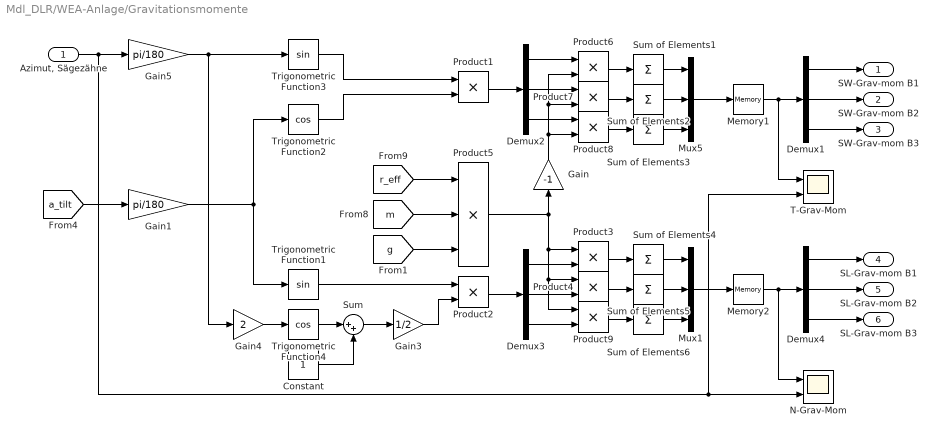
== system Mdl_DLR/WEA-Anlage/Gravitationsmomente ==
  "Azimut, Sägezähne" : Inport
  Constant : Constant
  Demux{1..4} (4 alike) : Demux  Outputs=3
  Gain : Gain  Gain=-1
  Gain1 : Gain  Gain=pi/180
  Gain3 : Gain  Gain=1/2
  Gain4 : Gain  Gain=2
  Gain5 : Gain  Gain=pi/180
  Memory1 : Memory
  Memory2 : Memory
  Mux1 : Mux  Inputs=3
  Mux5 : Mux  Inputs=3
  N-Grav-Mom : Scope  NumInputPorts=2
  Product{1..4,6..9} (8 alike) : Product  RndMeth=Zero
  Product5 : Product  Inputs=3  RndMeth=Zero
  Sum : Sum  Inputs=|++
  Sum of Elements{1..6} (6 alike) : Sum  Inputs=+
  T-Grav-Mom : Scope  NumInputPorts=2
  Trigonometric Function1 : Trigonometry
  Trigonometric Function2 : Trigonometry  Operator=cos
  Trigonometric Function3 : Trigonometry
  Trigonometric Function4 : Trigonometry  Operator=cos
  SW-Grav-mom B1 : Outport  VectorParamsAs1DForOutWhenUnconnected=off
  SW-Grav-mom B2 : Outport  Port=2  VectorParamsAs1DForOutWhenUnconnected=off
  SW-Grav-mom B3 : Outport  Port=3  VectorParamsAs1DForOutWhenUnconnected=off
  SL-Grav-mom B1 : Outport  Port=4  VectorParamsAs1DForOutWhenUnconnected=off
  SL-Grav-mom B2 : Outport  Port=5  VectorParamsAs1DForOutWhenUnconnected=off
  SL-Grav-mom B3 : Outport  Port=6  VectorParamsAs1DForOutWhenUnconnected=off
  wires:
  Gain5/1 -> Trigonometric Function3/1, Gain4/1
  Product5/1 -> Gain/1, Product3/1, Product4/1, Product9/1
  "Azimut, Sägezähne"/1 -> Gain5/1, N-Grav-Mom/2, T-Grav-Mom/2
  Memory1/1 -> Demux1/1, T-Grav-Mom/1
  Product6/1 -> Sum of Elements1/1
  Sum of Elements1/1 -> Mux5/1
  Product7/1 -> Sum of Elements2/1
  Product8/1 -> Sum of Elements3/1
  Sum of Elements2/1 -> Mux5/2
  Sum of Elements3/1 -> Mux5/3
  Demux2/1 -> Product6/1
  Demux2/2 -> Product7/1
  Demux2/3 -> Product8/1
  Mux5/1 -> Memory1/1
  [r_eff] -> Product5/1
  [m] -> Product5/2
  Demux1/1 -> SW-Grav-mom B1/1
  Demux1/2 -> SW-Grav-mom B2/1
  Demux1/3 -> SW-Grav-mom B3/1
  [g] -> Product5/3
  Gain/1 -> Product6/2, Product7/2, Product8/2
  Trigonometric Function4/1 -> Sum/1
  Sum/1 -> Gain3/1
  Constant/1 -> Sum/2
  Gain3/1 -> Product2/2
  [a_tilt] -> Gain1/1
  Gain1/1 -> Trigonometric Function2/1, Trigonometric Function1/1
  Trigonometric Function3/1 -> Product1/1
  Trigonometric Function2/1 -> Product1/2
  Product1/1 -> Demux2/1
  Gain4/1 -> Trigonometric Function4/1
  Trigonometric Function1/1 -> Product2/1
  Product2/1 -> Demux3/1
  Memory2/1 -> Demux4/1, N-Grav-Mom/1
  Product3/1 -> Sum of Elements4/1
  Sum of Elements4/1 -> Mux1/1
  Product4/1 -> Sum of Elements5/1
  Product9/1 -> Sum of Elements6/1
  Sum of Elements5/1 -> Mux1/2
  Sum of Elements6/1 -> Mux1/3
  Mux1/1 -> Memory2/1
  Demux4/1 -> SL-Grav-mom B1/1
  Demux4/2 -> SL-Grav-mom B2/1
  Demux4/3 -> SL-Grav-mom B3/1
  Demux3/3 -> Product9/2
  Demux3/2 -> Product4/2
  Demux3/1 -> Product3/2

== system Mdl_DLR/WEA-Anlage/Subsystem ==
  Pitch : Inport
  Add1 : Sum  Inputs=+-
  Add2 : Sum  Inputs=+-
  Add3 : Sum  Inputs=+-
  Demux : Demux  Outputs=3
  Gain : Gain  Gain=-1
  Gain1 : Gain  Gain=-1
  Mux : Mux  Inputs=3
  CPC +IPC : Outport  VectorParamsAs1DForOutWhenUnconnected=off
  theta : Outport  Port=2  VectorParamsAs1DForOutWhenUnconnected=off
  wires:
  [Verw] -> Gain/1  "Verw."
  Add1/1 -> Mux/1  "radialer Blattsteuerwinkel"
  Pitch/1 -> Gain1/1, Demux/1  "Pitch"
  Demux/1 -> Add1/2
  Demux/2 -> Add2/2
  Demux/3 -> Add3/2
  Add2/1 -> Mux/2  "radialer Blattsteuerwinkel"
  Add3/1 -> Mux/3  "radialer Blattsteuerwinkel"
  Mux/1 -> theta/1
  Gain/1 -> Add1/1, Add3/1, Add2/1
  Gain1/1 -> CPC +IPC/1

== system Mdl_DLR/WEA-Anlage/Sägezähne ==
  Azimut : Inport
  Add4 : Sum
  Add5 : Sum
  Azimute : Scope
  Gain4 : Gain  Gain=180/pi
  Gain6 : Gain  Gain=2
  Generator- moment1 : Constant  Value=-120
  Grad : Constant  Value=0
  Grad1 : Constant  Value=360
  Memory1 : Memory
  Memory2 : Memory
  Memory4 : Memory
  Mux4 : Mux  Inputs=3
  Sum2 : Sum  Inputs=|+-
  Sum3 : Sum  Inputs=|++
  Sum4 : Sum  Inputs=+|+
  Sum5 : Sum  Inputs=|+-
  Switch : Switch  Threshold=360
  Sägezähne : Outport  VectorParamsAs1DForOutWhenUnconnected=off
  wires:
  Grad/1 -> Switch/3
  Grad1/1 -> Switch/1
  Gain4/1 -> Sum2/1, Sum5/1, Memory4/1  "Azimut"
  Switch/1 -> Sum3/1
  Sum2/1 -> Memory1/1, Mux4/1, Add4/1, Add5/1  "Azimut"
  Sum3/1 -> Memory2/1, Sum2/2  "Omega"
  Memory2/1 -> Sum3/2
  Sum4/1 -> Switch/2
  Sum5/1 -> Sum4/2
  Memory4/1 -> Sum5/2
  Azimut/1 -> Gain4/1
  Memory1/1 -> Sum4/1
  Generator- moment1/1 -> Add4/2, Gain6/1
  Add4/1 -> Mux4/2
  Mux4/1 -> Sägezähne/1, Azimute/1  "Azimut"
  Add5/1 -> Mux4/3
  Gain6/1 -> Add5/2

== system Mdl_DLR/WEA-Anlage/WECS Tower Movement ==
  note: Tower Fore-Aft Motion
  note: Tower Side-By-Side Motion
  Aerodynamic Force [N] : Inport
  Aerodynamic Torque [Nm] : Inport  Port=2
  Gain : Gain  Gain=wecs.Btsw/wecs.mt
  Gain1 : Gain  Gain=wecs.Ktsw/wecs.mt
  Gain10 : Gain  Gain=3/(2*wecs.H)
  Gain{4,6,8,14} (4 alike) : Gain  Gain=DT
  Gain2 : Gain  Gain=wecs.Bt/wecs.mt
  Gain3 : Gain  Gain=wecs.Kt/wecs.mt
  Gain5 : Gain  Gain=1/wecs.mt
  Gain7 : Gain  Gain=1/wecs.mt
  Memory{1..4} (4 alike) : Memory
  Sum : Sum  Inputs=+--
  Sum{1,3..5} (4 alike) : Sum
  Sum2 : Sum  Inputs=+--
  xdotfa [m/s^2] : Outport  VectorParamsAs1DForOutWhenUnconnected=off
  xdotdotsw [m/s^2] : Outport  Port=2  VectorParamsAs1DForOutWhenUnconnected=off
  xdotdotfa [m/s^2] : Outport  Port=3  VectorParamsAs1DForOutWhenUnconnected=off
  wires:
  Memory4/1 -> Gain6/1, xdotfa [m/s^2]/1, Sum4/2, Gain2/1  "xdotfa"
  Sum2/1 -> Gain8/1, xdotdotfa [m/s^2]/1  "xdotdotfa"
  Gain5/1 -> Sum2/1
  Gain2/1 -> Sum2/3
  Memory2/1 -> Sum3/2, Gain3/1  "xfa"
  Gain3/1 -> Sum2/2
  Aerodynamic Force [N]/1 -> Gain5/1
  Gain/1 -> Sum/3
  Gain1/1 -> Sum/2
  Gain7/1 -> Sum/1
  Memory1/1 -> Gain/1, Sum1/2, Gain14/1  "xdotss"
  Memory3/1 -> Gain1/1, Sum5/2  "xss"
  Gain10/1 -> Gain7/1  "xdotdotss"
  Aerodynamic Torque [Nm]/1 -> Gain10/1
  Sum5/1 -> Memory3/1  "xdotdotss"
  Gain14/1 -> Sum5/1
  Sum/1 -> xdotdotsw [m/s^2]/1, Gain4/1  "xdotss"
  Sum1/1 -> Memory1/1  "xdotdotss"
  Gain4/1 -> Sum1/1
  Sum3/1 -> Memory2/1  "xdotdotss"
  Gain6/1 -> Sum3/1
  Gain8/1 -> Sum4/1
  Sum4/1 -> Memory4/1  "xdotdotss"

== system Mdl_DLR/WEA-Anlage/Abwindmodelle/vi-global ==
  Abs : Abs
  B1 : Constant  Value=100
  Divide : Product  Inputs=**/
  Divide1 : Product  Inputs=*/
  Divide2 : Product  Inputs=/*
  Divide3 : Product
  Gain : Gain  Gain=2
  Gain1 : Gain  Gain=pi
  Math Function : Math  Operator=square  SignedPower=on  SaturateOnIntegerOverflow=on
  Math Function1 : Math  Operator=sqrt  SignedPower=on  SaturateOnIntegerOverflow=on
  Math Function2 : Math  Operator=square  SignedPower=on  SaturateOnIntegerOverflow=on
  Math Function3 : Math  Operator=square  SignedPower=on  SaturateOnIntegerOverflow=on
  Memory5 : Memory
  Product : Product  Inputs=3  RndMeth=Zero
  Sign : Signum
  Sum : Sum  Inputs=|++
  Sum of Elements : Sum  Inputs=+
  Sum1 : Sum  Inputs=|+-
  Sum2 : Sum  Inputs=|+-
  ra/R : Constant  Value=0.1
  viG : Outport  VectorParamsAs1DForOutWhenUnconnected=off
  wires:
  Gain/1 -> Product/1
  Math Function/1 -> Gain1/1
  Gain1/1 -> Product/2
  Product/1 -> Divide/3
  Divide/1 -> Abs/1, Sign/1
  Sum of Elements/1 -> Divide/1
  [B] -> Sum2/2, Divide1/1
  B1/1 -> Divide1/2, Sum2/1, Divide2/1
  Divide1/1 -> Sum/1
  Sum/1 -> Math Function2/1
  Math Function2/1 -> Sum1/2
  Divide2/1 -> Math Function3/1
  Math Function3/1 -> Sum1/1
  Sum1/1 -> Product/3
  [nBl] -> Divide/2
  [N] -> Sum of Elements/1
  [rho] -> Gain/1
  [R] -> Math Function/1
  ra/R/1 -> Sum/2
  Sum2/1 -> Divide2/2
  Memory5/1 -> viG/1
  Abs/1 -> Math Function1/1
  Math Function1/1 -> Divide3/1
  Sign/1 -> Divide3/2
  Divide3/1 -> Memory5/1

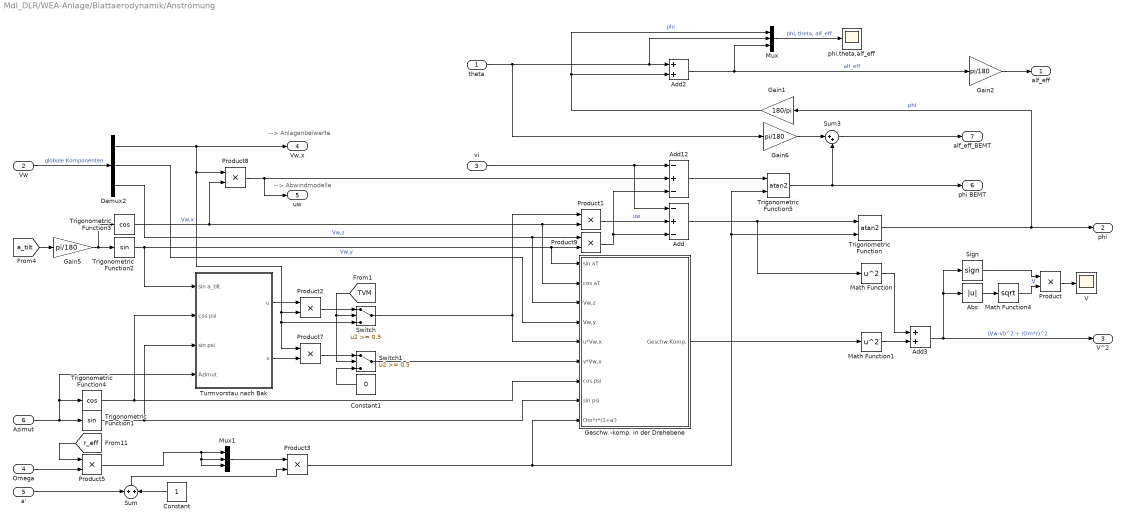
== system Mdl_DLR/WEA-Anlage/Blattaerodynamik/Anströmung ==
  note: --> Abwindmodelle
  note: --> Anlagenbeiwerte
  theta : Inport
  Vw : Inport  Port=2
  vi : Inport  Port=3
  Omega : Inport  Port=4
  a' : Inport  Port=5
  Azimut : Inport  Port=6
  Abs : Abs
  Add : Sum  Inputs=-+-
  Add12 : Sum  Inputs=-+-
  Add2 : Sum
  Add3 : Sum
  Constant : Constant
  Constant1 : Constant  Value=0
  Demux2 : Demux  Outputs=3
  Gain1 : Gain  Gain=180/pi
  Gain2 : Gain  Gain=pi/180
  Gain5 : Gain  Gain=pi/180
  Gain6 : Gain  Gain=pi/180
  Geschw.-komp. in der Drehebene : Subsystem
  Math Function : Math  Operator=square  SignedPower=on  SaturateOnIntegerOverflow=on
  Math Function1 : Math  Operator=square  SignedPower=on  SaturateOnIntegerOverflow=on
  Math Function4 : Math  Operator=sqrt  SignedPower=on  SaturateOnIntegerOverflow=on
  Mux : Mux  Inputs=3
  Mux1 : Mux  Inputs=3
  Product{,1..3,5,7..9} (8 alike) : Product  RndMeth=Zero
  Sign : Signum
  Sum : Sum  Inputs=+|+
  Sum3 : Sum  Inputs=|++
  Switch : Switch  Threshold=0.5
  Switch1 : Switch  Threshold=0.5
  Trigonometric Function : Trigonometry  Operator=atan2
  Trigonometric Function1 : Trigonometry
  Trigonometric Function2 : Trigonometry
  Trigonometric Function3 : Trigonometry  Operator=cos
  Trigonometric Function4 : Trigonometry  Operator=cos
  Trigonometric Function5 : Trigonometry  Operator=atan2
  Turmvorstau nach Bak : Subsystem
  V : Scope
  phi,theta,alf_eff : Scope
  alf_eff : Outport  VectorParamsAs1DForOutWhenUnconnected=off
  phi : Outport  Port=2  VectorParamsAs1DForOutWhenUnconnected=off
  V^2 : Outport  Port=3  VectorParamsAs1DForOutWhenUnconnected=off
  Vw,x : Outport  Port=4  VectorParamsAs1DForOutWhenUnconnected=off
  uw : Outport  Port=5  VectorParamsAs1DForOutWhenUnconnected=off
  phi BEMT : Outport  Port=6  VectorParamsAs1DForOutWhenUnconnected=off
  alf_eff_BEMT : Outport  Port=7  VectorParamsAs1DForOutWhenUnconnected=off
  wires:
  Trigonometric Function/1 -> Gain1/1, phi/1  "phi"
  Mux/1 -> phi,theta,alf_eff/1  "phi, theta, alf_eff"
  Gain1/1 -> Mux/1, Add2/2  "phi"
  Gain2/1 -> alf_eff/1
  Math Function1/1 -> Add3/2
  Math Function/1 -> Add3/1
  Add3/1 -> V^2/1, Abs/1, Sign/1  "(Vw-vi)^2 + (Om*r)^2"
  Math Function4/1 -> Product/2  "V"
  Add/1 -> Trigonometric Function/1, Math Function/1
  Omega/1 -> Product5/2
  [r_eff] -> Product5/1
  vi/1 -> Add/1, Add12/1
  Sum/1 -> Product3/2
  Abs/1 -> Math Function4/1
  Sign/1 -> Product/1
  Product/1 -> V/1
  Azimut/1 -> Trigonometric Function1/1, Trigonometric Function4/1, Turmvorstau nach Bak/4(Azimut)
  Trigonometric Function1/1 -> Turmvorstau nach Bak/3(sin psi), Geschw.-komp. in der Drehebene/8(sin psi)
  [a_tilt] -> Gain5/1
  Trigonometric Function2/1 -> Product9/2, Geschw.-komp. in der Drehebene/1(sin aT), Turmvorstau nach Bak/1(sin a_tilt)
  Gain5/1 -> Trigonometric Function2/1, Trigonometric Function3/1
  Trigonometric Function3/1 -> Product8/2, Product1/2, Geschw.-komp. in der Drehebene/2(cos aT)
  Product1/1 -> Add/2  "uw"
  Demux2/1 -> Vw,x/1, Product8/1, Product2/2, Product7/1, Switch/3  "Vw,x"
  Demux2/3 -> Product9/1, Geschw.-komp. in der Drehebene/3(Vw,z)  "Vw,z"
  Product9/1 -> Add/3, Add12/3
  Geschw.-komp. in der Drehebene/1(Geschw.Komp.) -> Math Function1/1
  Trigonometric Function4/1 -> Turmvorstau nach Bak/2(cos psi), Geschw.-komp. in der Drehebene/7(cos psi)
  Vw/1 -> Demux2/1  "globale Komponenten"
  Demux2/2 -> Geschw.-komp. in der Drehebene/4(Vw,y)  "Vw,y"
  Turmvorstau nach Bak/1(u) -> Product2/1
  Turmvorstau nach Bak/2(v) -> Product7/2
  Product8/1 -> uw/1, Add12/2
  Switch/1 -> Product1/1, Geschw.-komp. in der Drehebene/5(u*Vw,x)
  [TVM] -> Switch/2, Switch1/2
  Product2/1 -> Switch/1
  Product7/1 -> Switch1/1
  Constant1/1 -> Switch1/3
  Product3/1 -> Trigonometric Function/2, Trigonometric Function5/2, Geschw.-komp. in der Drehebene/9(Om*r*(1+a'))
  theta/1 -> Add2/1, Mux/2, Gain6/1
  Add2/1 -> Gain2/1, Mux/3  "alf_eff"
  Add12/1 -> Trigonometric Function5/1
  Trigonometric Function5/1 -> phi BEMT/1, Sum3/2
  Sum3/1 -> alf_eff_BEMT/1
  Switch1/1 -> Geschw.-komp. in der Drehebene/6(v*Vw,x)
  a'/1 -> Sum/1
  Constant/1 -> Sum/2
  Gain6/1 -> Sum3/1
  Mux1/1 -> Product3/1
  Product5/1 -> Mux1/3, Mux1/2, Mux1/1

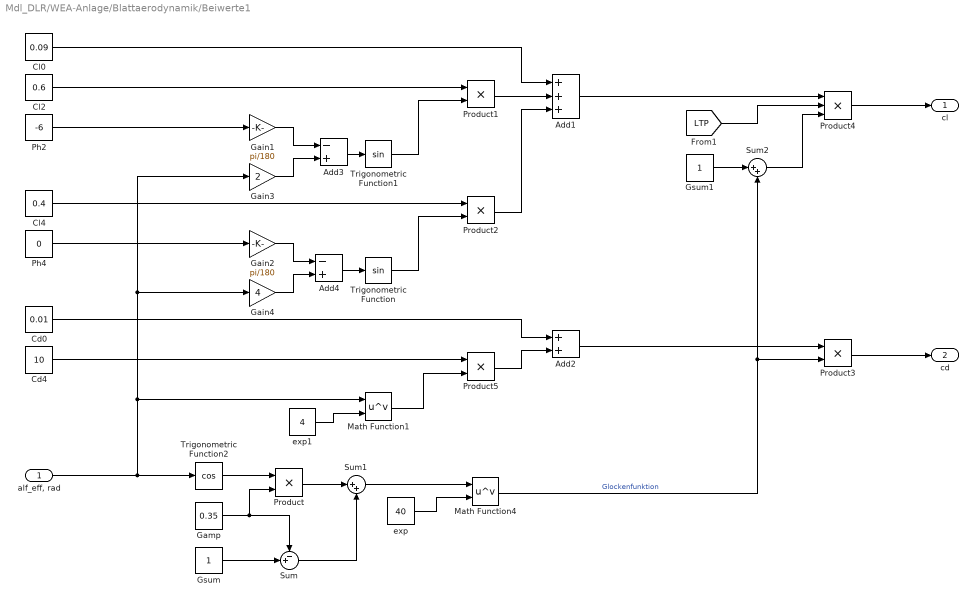
== system Mdl_DLR/WEA-Anlage/Blattaerodynamik/Beiwerte1 ==
  "alf_eff, rad" : Inport
  Add1 : Sum  Inputs=+++
  Add2 : Sum
  Add3 : Sum  Inputs=-+
  Add4 : Sum  Inputs=-+
  Cd0 : Constant  Value=0.01
  Cd4 : Constant  Value=10
  Cl0 : Constant  Value=0.09
  Cl2 : Constant  Value=0.6
  Cl4 : Constant  Value=0.4
  Gain1 : Gain  Gain=pi/180
  Gain2 : Gain  Gain=pi/180
  Gain3 : Gain  Gain=2
  Gain4 : Gain  Gain=4
  Gamp : Constant  Value=0.35
  Gsum : Constant
  Gsum1 : Constant
  Math Function1 : Math  Operator=pow  SignedPower=on  SaturateOnIntegerOverflow=on
  Math Function4 : Math  Operator=pow  SignedPower=on  SaturateOnIntegerOverflow=on
  Ph2 : Constant  Value=-6
  Ph4 : Constant  Value=0
  Product{,1..3,5} (5 alike) : Product  RndMeth=Zero
  Product4 : Product  Inputs=3  RndMeth=Zero
  Sum : Sum  Inputs=-+|
  Sum1 : Sum  Inputs=|++
  Sum2 : Sum  Inputs=|++
  Trigonometric Function : Trigonometry
  Trigonometric Function1 : Trigonometry
  Trigonometric Function2 : Trigonometry  Operator=cos
  exp : Constant  Value=40
  exp1 : Constant  Value=4
  cl : Outport  VectorParamsAs1DForOutWhenUnconnected=off
  cd : Outport  Port=2  VectorParamsAs1DForOutWhenUnconnected=off
  wires:
  [LTP] -> Product4/2
  Add2/1 -> Product3/1
  Product3/1 -> cd/1
  "alf_eff, rad"/1 -> Gain3/1, Gain4/1, Math Function1/1, Trigonometric Function2/1
  Product4/1 -> cl/1
  Add1/1 -> Product4/1
  Sum2/1 -> Product4/3
  Gsum1/1 -> Sum2/1
  Math Function4/1 -> Product3/2, Sum2/2  "Glockenfunktion"
  Sum1/1 -> Math Function4/1
  Product/1 -> Sum1/1
  Sum/1 -> Sum1/2
  Trigonometric Function2/1 -> Product/1
  Gamp/1 -> Product/2, Sum/1
  Gsum/1 -> Sum/2
  Product2/1 -> Add1/3
  Trigonometric Function/1 -> Product2/2
  Cl4/1 -> Product2/1
  Gain4/1 -> Add4/2
  Gain2/1 -> Add4/1
  Add4/1 -> Trigonometric Function/1
  Trigonometric Function1/1 -> Product1/2
  Cl2/1 -> Product1/1
  Add3/1 -> Trigonometric Function1/1
  Gain3/1 -> Add3/2
  Gain1/1 -> Add3/1
  Ph4/1 -> Gain2/1
  Ph2/1 -> Gain1/1
  Cl0/1 -> Add1/1
  Product1/1 -> Add1/2
  Cd0/1 -> Add2/1
  Cd4/1 -> Product5/1
  Product5/1 -> Add2/2
  Math Function1/1 -> Product5/2
  exp/1 -> Math Function4/2
  exp1/1 -> Math Function1/2

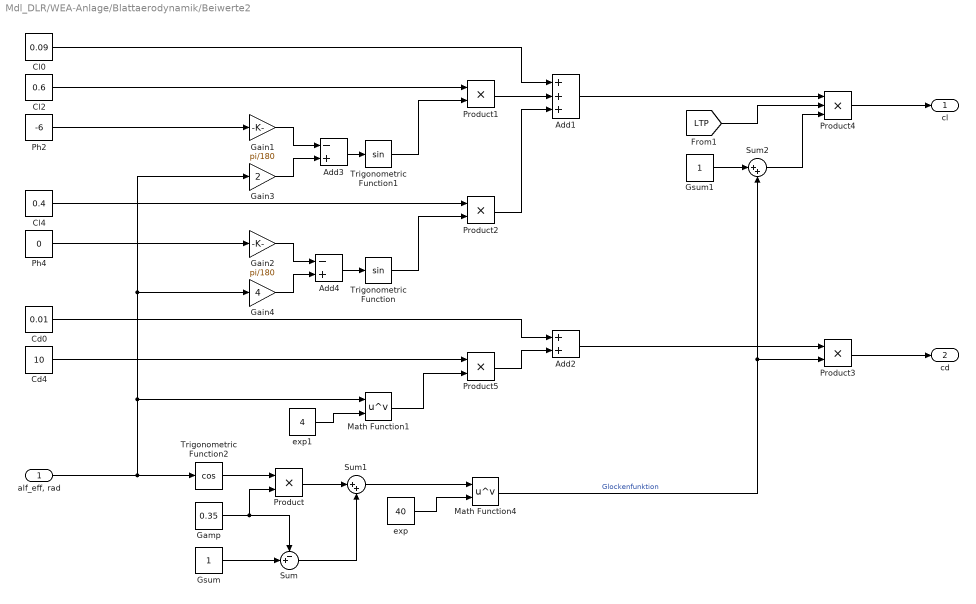
== system Mdl_DLR/WEA-Anlage/Blattaerodynamik/Beiwerte2 ==
  "alf_eff, rad" : Inport
  Add1 : Sum  Inputs=+++
  Add2 : Sum
  Add3 : Sum  Inputs=-+
  Add4 : Sum  Inputs=-+
  Cd0 : Constant  Value=0.01
  Cd4 : Constant  Value=10
  Cl0 : Constant  Value=0.09
  Cl2 : Constant  Value=0.6
  Cl4 : Constant  Value=0.4
  Gain1 : Gain  Gain=pi/180
  Gain2 : Gain  Gain=pi/180
  Gain3 : Gain  Gain=2
  Gain4 : Gain  Gain=4
  Gamp : Constant  Value=0.35
  Gsum : Constant
  Gsum1 : Constant
  Math Function1 : Math  Operator=pow  SignedPower=on  SaturateOnIntegerOverflow=on
  Math Function4 : Math  Operator=pow  SignedPower=on  SaturateOnIntegerOverflow=on
  Ph2 : Constant  Value=-6
  Ph4 : Constant  Value=0
  Product{,1..3,5} (5 alike) : Product  RndMeth=Zero
  Product4 : Product  Inputs=3  RndMeth=Zero
  Sum : Sum  Inputs=-+|
  Sum1 : Sum  Inputs=|++
  Sum2 : Sum  Inputs=|++
  Trigonometric Function : Trigonometry
  Trigonometric Function1 : Trigonometry
  Trigonometric Function2 : Trigonometry  Operator=cos
  exp : Constant  Value=40
  exp1 : Constant  Value=4
  cl : Outport  VectorParamsAs1DForOutWhenUnconnected=off
  cd : Outport  Port=2  VectorParamsAs1DForOutWhenUnconnected=off
  wires:
  exp1/1 -> Math Function1/2
  exp/1 -> Math Function4/2
  Math Function1/1 -> Product5/2
  Product5/1 -> Add2/2
  Cd4/1 -> Product5/1
  Cd0/1 -> Add2/1
  Product1/1 -> Add1/2
  Cl0/1 -> Add1/1
  Ph2/1 -> Gain1/1
  Ph4/1 -> Gain2/1
  Gain1/1 -> Add3/1
  Gain3/1 -> Add3/2
  Add3/1 -> Trigonometric Function1/1
  Cl2/1 -> Product1/1
  Trigonometric Function1/1 -> Product1/2
  Add4/1 -> Trigonometric Function/1
  Gain2/1 -> Add4/1
  Gain4/1 -> Add4/2
  Cl4/1 -> Product2/1
  Trigonometric Function/1 -> Product2/2
  Product2/1 -> Add1/3
  Gsum/1 -> Sum/2
  Gamp/1 -> Sum/1, Product/2
  Trigonometric Function2/1 -> Product/1
  Sum/1 -> Sum1/2
  Product/1 -> Sum1/1
  Sum1/1 -> Math Function4/1
  Math Function4/1 -> Sum2/2, Product3/2  "Glockenfunktion"
  Gsum1/1 -> Sum2/1
  Sum2/1 -> Product4/3
  Add1/1 -> Product4/1
  Product4/1 -> cl/1
  "alf_eff, rad"/1 -> Trigonometric Function2/1, Math Function1/1, Gain4/1, Gain3/1
  Product3/1 -> cd/1
  Add2/1 -> Product3/1
  [LTP] -> Product4/2

== system Mdl_DLR/WEA-Anlage/Blattaerodynamik/Blattbiegemomente ==
  T : Inport
  N : Inport  Port=2
  Demux : Demux  Outputs=3
  Demux1 : Demux  Outputs=3
  Mux1 : Mux  Inputs=3
  Mux5 : Mux  Inputs=3
  Product{1..6} (6 alike) : Product  RndMeth=Zero
  Sum of Elements{1..6} (6 alike) : Sum  Inputs=+
  SW-Aero-Mom : Outport  VectorParamsAs1DForOutWhenUnconnected=off
  SL-Aero-Mom : Outport  Port=2  VectorParamsAs1DForOutWhenUnconnected=off
  wires:
  Demux/1 -> Product1/1
  Demux/3 -> Product3/1
  Demux/2 -> Product2/1
  Product3/1 -> Sum of Elements2/1
  Product2/1 -> Sum of Elements1/1
  Product1/1 -> Sum of Elements4/1
  Sum of Elements4/1 -> Mux5/1
  Sum of Elements1/1 -> Mux5/2
  Sum of Elements2/1 -> Mux5/3
  [r_eff] -> Product1/2, Product2/2, Product3/2, Product4/2, Product5/2, Product6/2
  Demux1/1 -> Product4/1
  Demux1/3 -> Product6/1
  Demux1/2 -> Product5/1
  Product6/1 -> Sum of Elements5/1
  Product5/1 -> Sum of Elements3/1
  Product4/1 -> Sum of Elements6/1
  Sum of Elements6/1 -> Mux1/1
  Sum of Elements3/1 -> Mux1/2
  Sum of Elements5/1 -> Mux1/3
  Mux5/1 -> SW-Aero-Mom/1
  Mux1/1 -> SL-Aero-Mom/1
  N/1 -> Demux1/1
  T/1 -> Demux/1

== system Mdl_DLR/WEA-Anlage/Blattaerodynamik/Komponenten für BEMT ==
  "phi, BEMT" : Inport
  cl : Inport  Port=2
  cd : Inport  Port=3
  Produc1 : Product  RndMeth=Zero
  Product10 : Product  RndMeth=Zero
  Product12 : Product  RndMeth=Zero
  Product16 : Product  RndMeth=Zero
  Sum2 : Sum  Inputs=|+-
  Sum3 : Sum  Inputs=|++
  Trigonometric Function5 : Trigonometry  Operator=cos
  Trigonometric Function7 : Trigonometry
  sin phi : Outport  VectorParamsAs1DForOutWhenUnconnected=off
  cos phi : Outport  Port=2  VectorParamsAs1DForOutWhenUnconnected=off
  ct : Outport  Port=3  VectorParamsAs1DForOutWhenUnconnected=off
  cn : Outport  Port=4  VectorParamsAs1DForOutWhenUnconnected=off
  wires:
  Produc1/1 -> Sum2/2  "cos CD"
  Product16/1 -> Sum2/1  "sin CL"
  "phi, BEMT"/1 -> Trigonometric Function5/1, Trigonometric Function7/1
  Product12/1 -> Sum3/2  "sin CD"
  Product10/1 -> Sum3/1  "cos CL"
  cl/1 -> Product16/2, Product10/2
  cd/1 -> Produc1/2, Product12/2
  Sum2/1 -> ct/1  "Ct"
  Sum3/1 -> cn/1  "Cn"
  Trigonometric Function7/1 -> Product16/1, Product12/1, sin phi/1
  Trigonometric Function5/1 -> Produc1/1, Product10/1, cos phi/1

== system Mdl_DLR/WEA-Anlage/Blattaerodynamik/Normal-//Tangentialkraft ==
  cl : Inport
  cd : Inport  Port=2
  "phi, rad" : Inport  Port=3
  V^2 : Inport  Port=4
  Gain : Gain  Gain=1/2
  Mux : Mux  Inputs=3
  Mux1 : Mux  Inputs=3
  Produc : Product  RndMeth=Zero
  Product1 : Product  Inputs=4  RndMeth=Zero
  Product{2..8} (7 alike) : Product  RndMeth=Zero
  Sum : Sum  Inputs=|+-
  Sum1 : Sum  Inputs=|++
  Terminator : Terminator
  Terminator1 : Terminator
  Trigonometric Function1 : Trigonometry  Operator=cos
  Trigonometric Function3 : Trigonometry
  T : Outport  VectorParamsAs1DForOutWhenUnconnected=off
  N : Outport  Port=2  VectorParamsAs1DForOutWhenUnconnected=off
  tag scope: N=global
  wires:
  Produc/1 -> Sum/2  "cos CD"
  Product8/1 -> Sum/1  "sin CL"
  Gain/1 -> Product1/1
  V^2/1 -> Product1/2
  "phi, rad"/1 -> Trigonometric Function3/1, Trigonometric Function1/1
  [rho] -> Gain/1
  [c] -> Mux/2, Mux/1, Mux/3
  Product4/1 -> Sum1/2  "sin CD"
  Product2/1 -> Sum1/1  "cos CL"
  cl/1 -> Product6/1, Product8/2, Product2/2  "cl"
  cd/1 -> Product5/1, Produc/2, Product4/2  "cd"
  Sum/1 -> Product3/1  "Ct"
  Sum1/1 -> Product7/1  "Cn"
  Product3/1 -> T/1  "Tangential"
  Product7/1 -> N/1, [N]  "Normal"
  Product6/1 -> Terminator/1  "Lift"
  Product5/1 -> Terminator1/1  "Drag"
  Product1/1 -> Product5/2, Product6/2, Product7/2, Product3/2
  Mux/1 -> Product1/4
  [dr] -> Mux1/2, Mux1/1, Mux1/3
  Mux1/1 -> Product1/3
  Trigonometric Function3/1 -> Product8/1, Product4/1
  Trigonometric Function1/1 -> Produc/1, Product2/1
